simulink model "HexaMotor_V03"  (R2026a)
settings: Solver=FixedStepAuto  StopTime=inf  FixedStep=0.002  EnableMultiTasking=on
libraries: arduinolib x4, arduinosensorlib x1
settings Model: SILPILModeSetting=veronly  ExtModeTrigDuration=2  Creator=arkad  LastModifiedBy=arkad
settings HardwareCC: ProdLargestAtomicInteger=Long  ProdLargestAtomicFloat=Double  ProdHWDeviceType=ARM Compatible->ARM Cortex
settings RTWCC: SystemTargetFile=ert.tlc  HardwareBoard=Arduino Uno R4 Minima  TLCOptions=-aInlineSetEventsForThisBaseRateFcn=TLC_FALSE -aSuppressMultiTaskScheduler=TLC_FALSE -aRateBasedStepFcn=1  Toolchain=Arduino ARM M4  BuildConfiguration=Faster Runs  Description=Embedded Coder
settings ERTTargetCC: ExtModeTransport=3.0  ExtModeAutomaticAllocSize=off  ExtModeStaticAllocSize=8192.0  SupportContinuousTime=on  SupportVariableSizeSignals=on

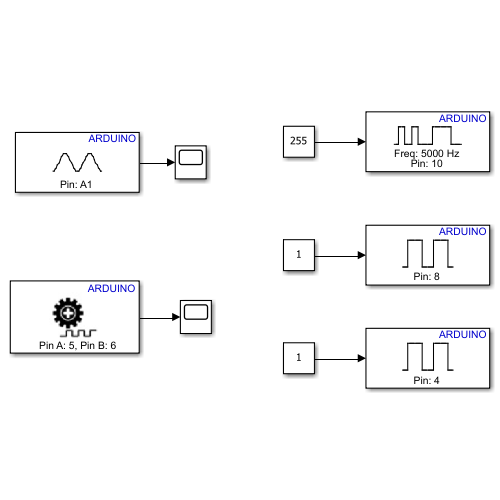
[thumbnail: Simulink's stored preview of the top-level diagram]
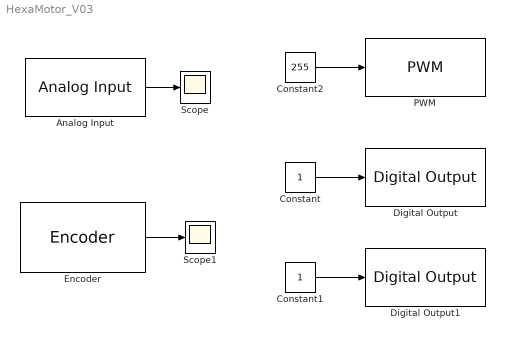
== system HexaMotor_V03 ==
  Analog Input : arduinolib/Analog Input  pinNumber=1  ReadResultsOnly=off  ConversionTriggerSource=Software  ExternalTriggerType=uint32( 0 )  OutputDataType=uint16  EnableConversionCompleteNotify=off  EnableOuputStatus=off  SampleTime=-1  blockPlatform=arduino
      settings: LibrarySourceBlock=gizmoLibrary/Arduino Utilities/Analog Input
  Constant : Constant
  Constant1 : Constant
  Constant2 : Constant  Value=255
  Digital Output : arduinolib/Digital Output  pinNumber=8  Direction=output  blockPlatform=arduino
      settings: LibrarySourceBlock=gizmoLibrary/Arduino Utilities/Digital Output
  Digital Output1 : arduinolib/Digital Output  pinNumber=4  Direction=output  blockPlatform=arduino
      settings: LibrarySourceBlock=gizmoLibrary/Arduino Utilities/Digital Output
  Encoder : arduinosensorlib/Encoder  InputA=5  InputB=6  Mode=No reset  SampleTime=-1
  PWM : arduinolib/PWM  pinNumber=10  frequencyType=Specify  desiredFrequency=5000  achievableFrequency=5000
      settings: LibrarySourceBlock=gizmoLibrary/Arduino Utilities/PWM
  Scope : Scope
      settings: ActiveDisplayYMinimum=-511.87499999999989  ActiveDisplayYMaximum=4606.875
  Scope1 : Scope
      settings: ActiveDisplayYMinimum=-9.125  ActiveDisplayYMaximum=-7.875
  wires:
  Analog Input/1 -> Scope/1
  Encoder/1 -> Scope1/1
  Constant/1 -> Digital Output/1
  Constant1/1 -> Digital Output1/1
  Constant2/1 -> PWM/1
